simulink model "popytka"  (R2018b)
settings: Solver=ode45  StartTime=0.0  StopTime=10.0  RelTol=1e-3  EnableMultiTasking=on
settings Model: Creator=bukova.2018  LastModifiedBy=Kirill
settings DataIOCC: LimitDataPoints=on  SaveFormat=Array  SignalLoggingSaveFormat=ModelDataLogs
settings OptimizationCC: ExpressionDepthLimit=2147483647  LifeSpan=inf
settings DebuggingCC: UnderspecifiedInitializationDetection=Classic  MergeDetectMultiDrivingBlocksExec=none  SolverPrmCheckMsg=warning  FcnCallInpInsideContextMsg=warning  StateNameClashWarn=warning  SFUnexpectedBacktrackingDiag=warning  SFNoUnconditionalDefaultTransitionDiag=warning  SFExecutionAtInitializationDiag=none
settings HardwareCC: ProdBitPerPointer=32  ProdBitPerSizeT=32  ProdBitPerPtrDiffT=32  ProdLargestAtomicFloat=None  ProdIntDivRoundTo=Undefined  ProdEndianess=Unspecified  ProdWordSize=32  ProdHWDeviceType=32-bit Generic
settings ModelReferenceCC: PropagateSignalLabelsOutOfModel=off
settings SFSimCC: SimUseLocalCustomCode=off
settings RTWCC: RTWUseLocalCustomCode=off
settings CodeAppCC: StateflowObjectComments=on
settings GRTTargetCC: TargetLangStandard=C89/C90 (ANSI)  GeneratePreprocessorConditionals=Disable all  CombineOutputUpdateFcns=off  GRTInterface=on
settings ConfigComp: CovMetricSettings=dw  CovHtmlReporting=on  CovSaveCumulativeToWorkspaceVar=on  CovSaveSingleToWorkspaceVar=on  CovExternalEMLEnable=off

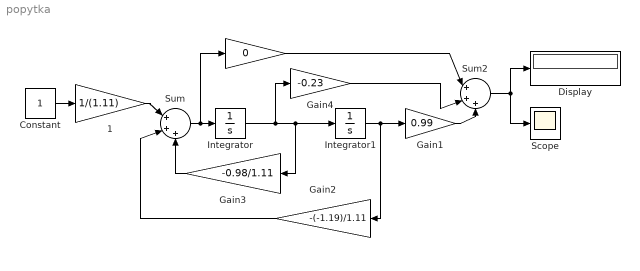
== system popytka ==
  " " : Gain  Gain=0
  " 1" : Gain  Gain=1/(1.11)
  Constant : Constant
  Display : Display
  Gain1 : Gain  Gain=0.99
  Gain2 : Gain  Gain=-(-1.19)/1.11
  Gain3 : Gain  Gain=-0.98/1.11
  Gain4 : Gain  Gain=-0.23
  Integrator : Integrator
  Integrator1 : Integrator
  Scope : Scope
  Sum : Sum  Inputs=|+++
  Sum2 : Sum  Inputs=|+++
  wires:
  Sum/1 -> Integrator/1, " "/1
  Integrator1/1 -> Gain1/1, Gain2/1
  Gain1/1 -> Sum2/3
  Integrator/1 -> Integrator1/1, Gain3/1, Gain4/1
  Gain2/1 -> Sum/2
  Gain3/1 -> Sum/3
  " "/1 -> Sum2/1
  Gain4/1 -> Sum2/2
  Constant/1 -> " 1"/1
  Sum2/1 -> Scope/1, Display/1
  " 1"/1 -> Sum/1
